simulink model "Mdl_Airbag"  (R2024b)
settings: Solver=FixedStepDiscrete  StartTime=0.0  StopTime=10.0  FixedStep=0.1  RelTol=1e-3  EnableMultiTasking=on
values from neighbouring files (symbols this model uses):
  CAN_AIRBAG_SIGN_ONE_VALUE = mpt.Parameter    [Mdl_Airbag_DD.m]
  CAN_AIRBAG_SIGN_TWO_VALUE = mpt.Parameter    [Mdl_Airbag_DD.m]
  CAN_AIRBAG_SIGN_ZERO_VALUE = mpt.Parameter    [Mdl_Airbag_DD.m]
undefined symbols (not defined in the file or in its folder): CLUSTER_INACTIVE, eAirbagIn, eSIGNAL_MISSING, eSIGNAL_NEVER_RECEIVED, IgnOff, NETWORK_NORMAL, tRxSafeSignalId_type_instance, tRxSafeSignalStatus_type_instance, TT_TURN_OFF, TT_TURN_ON
settings Model: Creator=AELANGO6  LastModifiedBy=AELANGO6
settings DataIOCC: SaveOutput=off
settings OptimizationCC: DefaultParameterBehavior=Inlined  EnhancedBackFolding=on  PassReuseOutputArgsAs=Individual arguments  ZeroExternalMemoryAtStartup=off  ZeroInternalMemoryAtStartup=off  MaxStackSize=750  RemoveLocalVariableInitialization=off  OptimizeBlockOrder=speed  DifferentSizesBufferReuse=on  OptimizationCustomize=off  EfficientTunableParamExpr=on
settings DebuggingCC: ParameterTunabilityLossMsg=error
settings SFSimCC: MATLABDynamicMemAlloc=off
settings RTWCC: Description=AUTOSAR  SystemTargetFile=autosar.tlc  GenCodeOnly=on  TemplateMakefile=ert_default_tmf  PortableWordSizes=on  DataTypeReplacement=CDataTypesFixedWidth
settings CodeAppCC: ForceParamTrailComments=on  IgnoreCustomStorageClasses=off  OperatorAnnotations=on  SimulinkDataObjDesc=on  SFDataObjDesc=on  InsertBlockDesc=on
settings STFCustomTargetCC: TargetLangStandard=C99 (ISO)  MultiwordLength=256  ParMdlRefBuildCompliant=on  CompOptLevelCompliant=on  IncludeMdlTerminateFcn=off  CombineOutputUpdateFcns=on  SuppressErrorStatus=on  ERTCustomFileBanners=on  SupportNonFinite=off  SupportComplex=off  SupportContinuousTime=off  SupportNonInlinedSFcns=off  RemoveResetFunc=on  ParenthesesLevel=Maximum  CastingMode=Standards  MATLABClassNameForMDSCustomization=Simulink.SoftwareTarget.ERTCustomization  AutosarCompliant=on  UseToolchainInfoCompliant=on  LookupTableObjectStructAxisOrder=2,1,3,4,...  LUTObjectStructOrderEvenSpacing=Size,Table,Breakpoints  SystemTargetFile=autosar.tlc
settings ERTTargetCC: TargetLangStandard=C99 (ISO)  ConcurrentExecutionCompliant=off  IncludeMdlTerminateFcn=off  SuppressErrorStatus=on  SupportNonFinite=off  SupportComplex=off  ParenthesesLevel=Maximum  CastingMode=Standards  ModelStepFunctionPrototypeControlCompliant=off  CPPClassGenCompliant=off  AutosarCompliant=on  LookupTableObjectStructAxisOrder=2,1,3,4,...  LUTObjectStructOrderEvenSpacing=Size,Table,Breakpoints  ERTCustomFileTemplate=example_file_process.tlc  ERTFilePackagingFormat=CompactWithDataFile  BooleanTrueId=TRUE  BooleanFalseId=FALSE

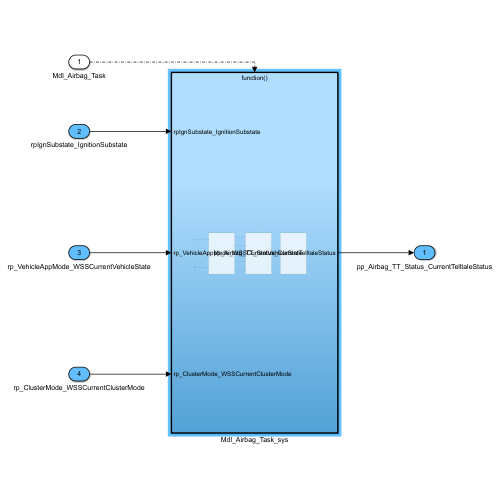
[thumbnail: Simulink's stored preview of the top-level diagram]
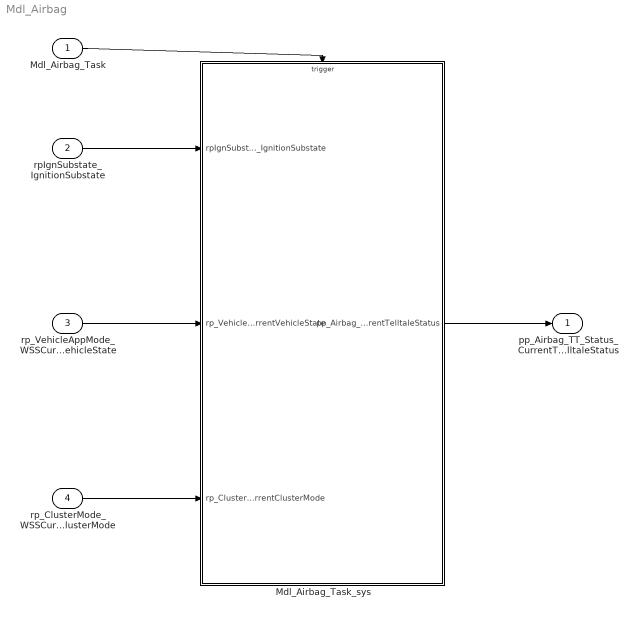
== system Mdl_Airbag ==
  Mdl_Airbag_Task : Inport  SampleTime=0.1  OutputFunctionCall=on
  rpIgnSubstate_IgnitionSubstate : Inport  Port=2  OutDataTypeStr=IgntionSubstateType  PortDimensions=1
  rp_VehicleAppMode_WSSCurrentVehicleState : Inport  Port=3  OutDataTypeStr=VehicleActiveModes  PortDimensions=1
  rp_ClusterMode_WSSCurrentClusterMode : Inport  Port=4  OutDataTypeStr=ClusterModes  PortDimensions=1
  Mdl_Airbag_Task_sys : Subsystem  TreatAsAtomicUnit=on
  pp_Airbag_TT_Status_CurrentTelltaleStatus : Outport  OutDataTypeStr=TT_OP_STATES
  wires:
  Mdl_Airbag_Task/1 -> Mdl_Airbag_Task_sys/Trigger
  Mdl_Airbag_Task_sys/1(pp_Airbag_TT_Status_CurrentTelltaleStatus) -> pp_Airbag_TT_Status_CurrentTelltaleStatus/1
  rp_VehicleAppMode_WSSCurrentVehicleState/1 -> Mdl_Airbag_Task_sys/2(rp_VehicleAppMode_WSSCurrentVehicleState)
  rpIgnSubstate_IgnitionSubstate/1 -> Mdl_Airbag_Task_sys/1(rpIgnSubstate_IgnitionSubstate)
  rp_ClusterMode_WSSCurrentClusterMode/1 -> Mdl_Airbag_Task_sys/3(rp_ClusterMode_WSSCurrentClusterMode)

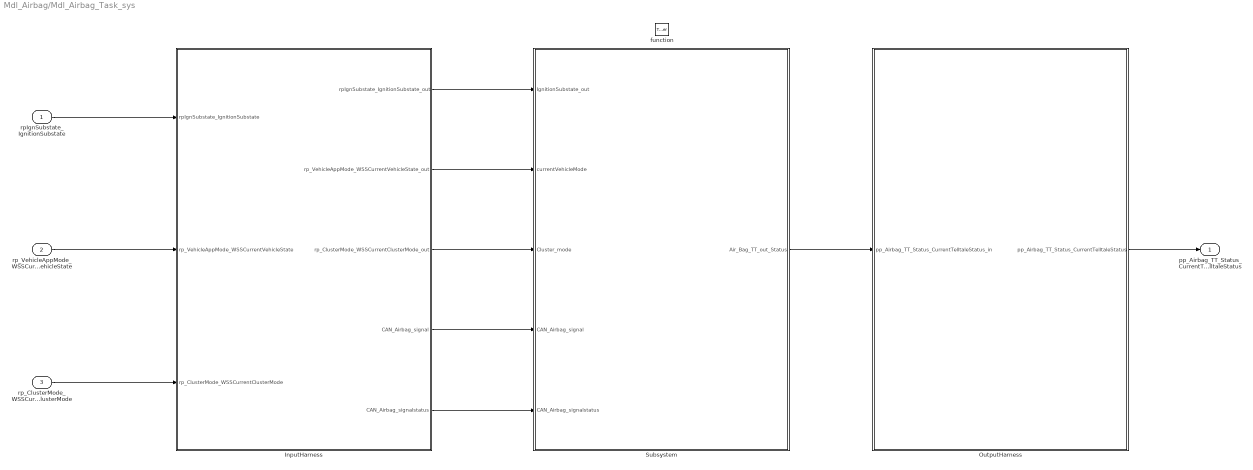
== system Mdl_Airbag/Mdl_Airbag_Task_sys ==
  rpIgnSubstate_IgnitionSubstate : Inport  OutDataTypeStr=IgntionSubstateType  PortDimensions=1
  rp_VehicleAppMode_WSSCurrentVehicleState : Inport  Port=2  OutDataTypeStr=VehicleActiveModes  PortDimensions=1
  rp_ClusterMode_WSSCurrentClusterMode : Inport  Port=3  OutDataTypeStr=ClusterModes  PortDimensions=1
  function : TriggerPort  TriggerType=function-call  VariantControl=(inherit)  SampleTimeType=periodic  SampleTime=-1
  InputHarness : Subsystem  Variant=on
  OutputHarness : Subsystem  Variant=on
  Subsystem : Subsystem
  pp_Airbag_TT_Status_CurrentTelltaleStatus : Outport  OutDataTypeStr=TT_OP_STATES  PortDimensions=1
  wires:
  rpIgnSubstate_IgnitionSubstate/1 -> InputHarness/1(rpIgnSubstate_IgnitionSubstate)
  rp_VehicleAppMode_WSSCurrentVehicleState/1 -> InputHarness/2(rp_VehicleAppMode_WSSCurrentVehicleState)
  rp_ClusterMode_WSSCurrentClusterMode/1 -> InputHarness/3(rp_ClusterMode_WSSCurrentClusterMode)
  Subsystem/1(Air_Bag_TT_out_Status) -> OutputHarness/1(pp_Airbag_TT_Status_CurrentTelltaleStatus_in)
  InputHarness/1(rpIgnSubstate_IgnitionSubstate_out) -> Subsystem/1(IgnitionSubstate_out)
  InputHarness/2(rp_VehicleAppMode_WSSCurrentVehicleState_out) -> Subsystem/2(currentVehicleMode)
  InputHarness/3(rp_ClusterMode_WSSCurrentClusterMode_out) -> Subsystem/3(Cluster_mode)
  InputHarness/4(CAN_Airbag_signal) -> Subsystem/4(CAN_Airbag_signal)
  InputHarness/5(CAN_Airbag_signalstatus) -> Subsystem/5(CAN_Airbag_signalstatus)
  OutputHarness/1(pp_Airbag_TT_Status_CurrentTelltaleStatus) -> pp_Airbag_TT_Status_CurrentTelltaleStatus/1

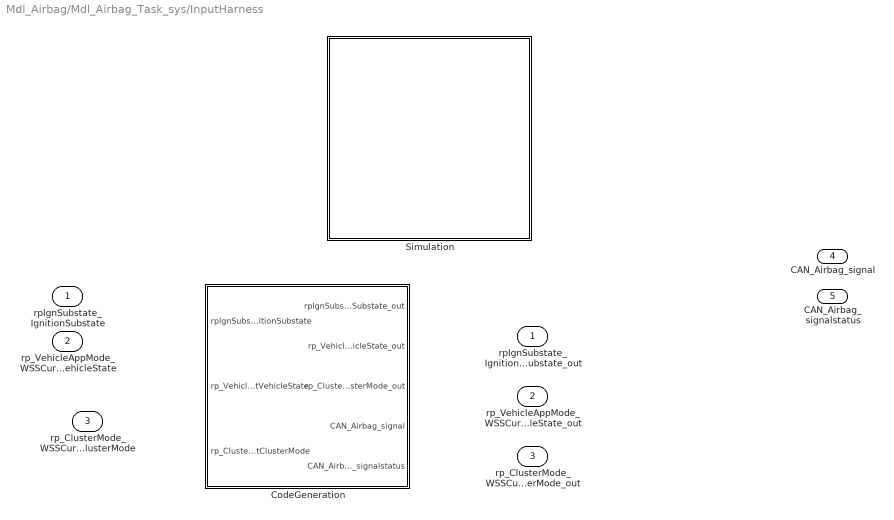
== system Mdl_Airbag/Mdl_Airbag_Task_sys/InputHarness ==
  rpIgnSubstate_IgnitionSubstate : Inport  OutDataTypeStr=IgntionSubstateType  PortDimensions=1
  rp_VehicleAppMode_WSSCurrentVehicleState : Inport  Port=2  OutDataTypeStr=VehicleActiveModes  PortDimensions=1
  rp_ClusterMode_WSSCurrentClusterMode : Inport  Port=3  OutDataTypeStr=ClusterModes  PortDimensions=1
  CodeGeneration : Subsystem  VariantControl=CODEGENERATION
  Simulation : Subsystem  VariantControl=SIMULATION
  rpIgnSubstate_IgnitionSubstate_out : Outport  OutDataTypeStr=IgntionSubstateType  PortDimensions=1
  rp_VehicleAppMode_WSSCurrentVehicleState_out : Outport  Port=2  OutDataTypeStr=VehicleActiveModes  PortDimensions=1
  rp_ClusterMode_WSSCurrentClusterMode_out : Outport  Port=3  OutDataTypeStr=ClusterModes  PortDimensions=1
  CAN_Airbag_signal : Outport  Port=4  VectorParamsAs1DForOutWhenUnconnected=off
  CAN_Airbag_signalstatus : Outport  Port=5  VectorParamsAs1DForOutWhenUnconnected=off

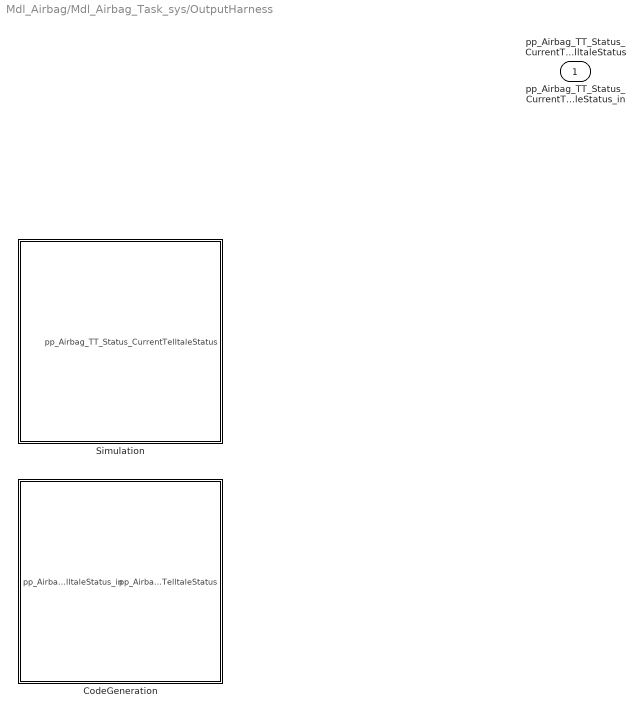
== system Mdl_Airbag/Mdl_Airbag_Task_sys/OutputHarness ==
  pp_Airbag_TT_Status_CurrentTelltaleStatus_in : Inport  OutDataTypeStr=TT_OP_STATES  PortDimensions=1
  CodeGeneration : Subsystem  VariantControl=CODEGENERATION
  Simulation : Subsystem  VariantControl=SIMULATION
  pp_Airbag_TT_Status_CurrentTelltaleStatus : Outport  OutDataTypeStr=TT_OP_STATES  PortDimensions=1

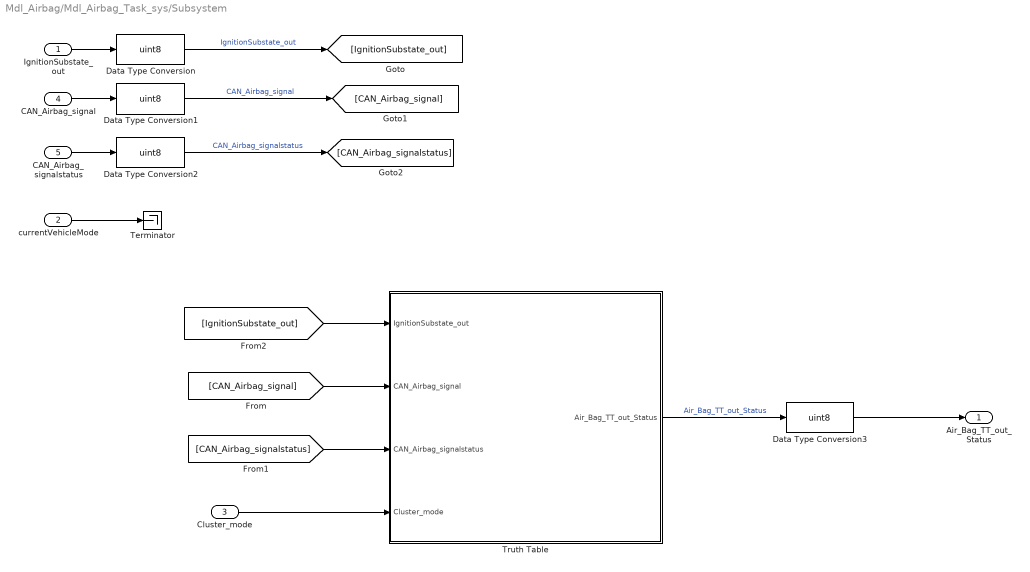
== system Mdl_Airbag/Mdl_Airbag_Task_sys/Subsystem ==
  IgnitionSubstate_out : Inport
  currentVehicleMode : Inport  Port=2
  Cluster_mode : Inport  Port=3
  CAN_Airbag_signal : Inport  Port=4
  CAN_Airbag_signalstatus : Inport  Port=5
  Data Type Conversion{,1..3} (4 alike) : DataTypeConversion  OutDataTypeStr=uint8  SaturateOnIntegerOverflow=off  RndMeth=Floor
  Terminator : Terminator
  Truth Table : Truth Table  TreatAsAtomicUnit=on
  Air_Bag_TT_out_Status : Outport  VectorParamsAs1DForOutWhenUnconnected=off
  wires:
  CAN_Airbag_signal/1 -> Data Type Conversion1/1
  CAN_Airbag_signalstatus/1 -> Data Type Conversion2/1
  IgnitionSubstate_out/1 -> Data Type Conversion/1
  Data Type Conversion/1 -> [IgnitionSubstate_out]  "IgnitionSubstate_out"
  Data Type Conversion1/1 -> [CAN_Airbag_signal]  "CAN_Airbag_signal"
  Data Type Conversion2/1 -> [CAN_Airbag_signalstatus]  "CAN_Airbag_signalstatus"
  [IgnitionSubstate_out] -> Truth Table/1(IgnitionSubstate_out)
  [CAN_Airbag_signal] -> Truth Table/2(CAN_Airbag_signal)
  [CAN_Airbag_signalstatus] -> Truth Table/3(CAN_Airbag_signalstatus)
  Truth Table/1(Air_Bag_TT_out_Status) -> Data Type Conversion3/1  "Air_Bag_TT_out_Status"
  Data Type Conversion3/1 -> Air_Bag_TT_out_Status/1
  Cluster_mode/1 -> Truth Table/4(Cluster_mode)
  currentVehicleMode/1 -> Terminator/1

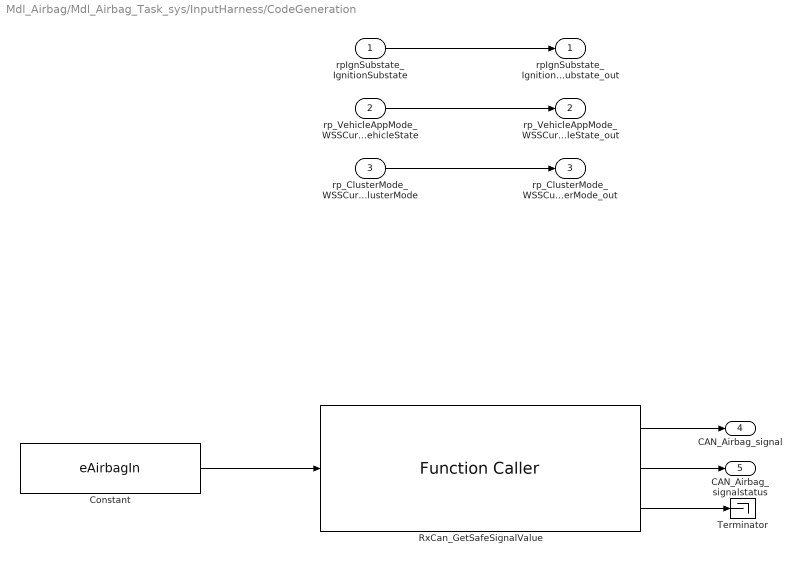
== system Mdl_Airbag/Mdl_Airbag_Task_sys/InputHarness/CodeGeneration ==
  rpIgnSubstate_IgnitionSubstate : Inport  OutDataTypeStr=IgntionSubstateType  PortDimensions=1
  rp_VehicleAppMode_WSSCurrentVehicleState : Inport  Port=2  OutDataTypeStr=VehicleActiveModes  PortDimensions=1
  rp_ClusterMode_WSSCurrentClusterMode : Inport  Port=3  OutDataTypeStr=ClusterModes  PortDimensions=1
  Constant : Constant  Value=eAirbagIn
  RxCan_GetSafeSignalValue : FunctionCaller  FunctionPrototype=[pSignalValue,pSignalStatus,error_status] = RxCan_GetSafeSignalValue(SignalId)  InputArgumentSpecifications=tRxSafeSignalId_type_instance(1)  OutputArgumentSpecifications=uint8(1) ,tRxSafeSignalStatus_type_instance(1) ,uint8(1)
  Terminator : Terminator
  rpIgnSubstate_IgnitionSubstate_out : Outport  OutDataTypeStr=IgntionSubstateType  PortDimensions=1
  rp_VehicleAppMode_WSSCurrentVehicleState_out : Outport  Port=2  OutDataTypeStr=VehicleActiveModes  PortDimensions=1
  rp_ClusterMode_WSSCurrentClusterMode_out : Outport  Port=3  OutDataTypeStr=ClusterModes  PortDimensions=1
  CAN_Airbag_signal : Outport  Port=4  VectorParamsAs1DForOutWhenUnconnected=off
  CAN_Airbag_signalstatus : Outport  Port=5  VectorParamsAs1DForOutWhenUnconnected=off
  wires:
  rpIgnSubstate_IgnitionSubstate/1 -> rpIgnSubstate_IgnitionSubstate_out/1
  rp_VehicleAppMode_WSSCurrentVehicleState/1 -> rp_VehicleAppMode_WSSCurrentVehicleState_out/1
  rp_ClusterMode_WSSCurrentClusterMode/1 -> rp_ClusterMode_WSSCurrentClusterMode_out/1
  RxCan_GetSafeSignalValue/2 -> CAN_Airbag_signalstatus/1
  RxCan_GetSafeSignalValue/3 -> Terminator/1
  RxCan_GetSafeSignalValue/1 -> CAN_Airbag_signal/1
  Constant/1 -> RxCan_GetSafeSignalValue/1

== system Mdl_Airbag/Mdl_Airbag_Task_sys/InputHarness/Simulation ==

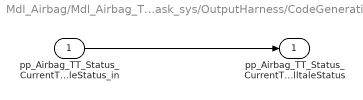
== system Mdl_Airbag/Mdl_Airbag_Task_sys/OutputHarness/CodeGeneration ==
  pp_Airbag_TT_Status_CurrentTelltaleStatus_in : Inport  OutDataTypeStr=TT_OP_STATES  PortDimensions=1
  pp_Airbag_TT_Status_CurrentTelltaleStatus : Outport  OutDataTypeStr=TT_OP_STATES  PortDimensions=1
  wires:
  pp_Airbag_TT_Status_CurrentTelltaleStatus_in/1 -> pp_Airbag_TT_Status_CurrentTelltaleStatus/1

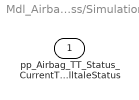
== system Mdl_Airbag/Mdl_Airbag_Task_sys/OutputHarness/Simulation ==
  pp_Airbag_TT_Status_CurrentTelltaleStatus : Outport  OutDataTypeStr=TT_OP_STATES  PortDimensions=1

== matlab function Mdl_Airbag/Mdl_Airbag_Task_sys/Subsystem/Truth Table ==
  data: IgnitionSubstate_out input; Air_Bag_TT_out_Status output; CAN_Airbag_signal input; CAN_Airbag_signalstatus input; CAN_AIRBAG_SIGN_ONE_VALUE parameter; CAN_AIRBAG_SIGN_TWO_VALUE parameter; CAN_AIRBAG_SIGN_ZERO_VALUE parameter; eSIGNAL_MISSING parameter; eSIGNAL_NEVER_RECEIVED parameter; IgnOff parameter; TT_TURN_ON parameter; TT_TURN_OFF parameter; NETWORK_NORMAL parameter; CLUSTER_INACTIVE parameter; Cluster_mode input
function Air_Bag_TT_out_Status = fcn(IgnitionSubstate_out, CAN_Airbag_signal, CAN_Airbag_signalstatus, CAN_AIRBAG_SIGN_ONE_VALUE, CAN_AIRBAG_SIGN_TWO_VALUE, CAN_AIRBAG_SIGN_ZERO_VALUE, eSIGNAL_MISSING, eSIGNAL_NEVER_RECEIVED, IgnOff, TT_TURN_ON, TT_TURN_OFF, NETWORK_NORMAL, CLUSTER_INACTIVE, Cluster_mode)

aVarTruthTableCondition_1 = false;
aVarTruthTableCondition_2 = false;


% Cluster Inactive , IGN Off Condition and Never Recvd condition

aVarTruthTableCondition_1 = logical((Cluster_mode == CLUSTER_INACTIVE) || (IgnitionSubstate_out == IgnOff) || (CAN_Airbag_signalstatus == eSIGNAL_NEVER_RECEIVED));

% Normal CAN Condition, Missing Condition

aVarTruthTableCondition_2 = logical((CAN_Airbag_signal ==CAN_AIRBAG_SIGN_ONE_VALUE) || (CAN_Airbag_signal == CAN_AIRBAG_SIGN_TWO_VALUE) || (CAN_Airbag_signalstatus == eSIGNAL_MISSING));

if (aVarTruthTableCondition_1)
    aFcnTruthTableAction_1();
elseif (aVarTruthTableCondition_2)
    aFcnTruthTableAction_2();
else % Default
    aFcnTruthTableAction_1();
end

function aFcnTruthTableAction_1()

% AirBag TT OFF Status

Air_Bag_TT_out_Status = TT_TURN_OFF;

function aFcnTruthTableAction_2()

% AirBag TT ON Status

Air_Bag_TT_out_Status = TT_TURN_ON;
